simulink model "ClimbSim"  (R2022a)
settings: Solver=VariableStepAuto  StartTime=0.0  StopTime=inf  RelTol=1e-3
values from neighbouring files (symbols this model uses):
  EMFCoefCim = 18.803/1000    (= 0.018803)    [Climbing.m]    (also in Launch.m; Launching.m)
  InputClimbing = 1    [Climbing.m]    (also in Launching.m)
  loadInertiaClimbing = 6.12 / (2*12.75) + (1.27*0.6*(0.0254^2))/2    (= 0.24024580596)    [Climbing.m]    (also in Launching.m)
  LVDTGain = 0.0084*1000    (= 8.4)    [Climbing.m]
  LVDTOffset = 0.0105    [Climbing.m]
  mechDampingConstantClimbing = (TorqueCoefCim * EMFCoefCim) / TerminalResistanceCim    (= 0.000117850936333)    [Climbing.m]    (also in Launching.m)
  TerminalInductanceCim = 122/1000000    (= 0.000122)    [Climbing.m]    (also in Launch.m; Launching.m)
  TerminalResistanceCim = 3    [Climbing.m]    (also in Launch.m; Launching.m)
  TorqueCoefCim = 18.803/1000    (= 0.018803)    [Climbing.m]    (also in Launch.m; Launching.m)
  TorqueDisturbanceClimb = 0    [Climbing.m]
libraries: slpidlib x1
settings Model: PacingRate=1.100000  Creator=JD Herlehy  LastModifiedBy=JD Herlehy

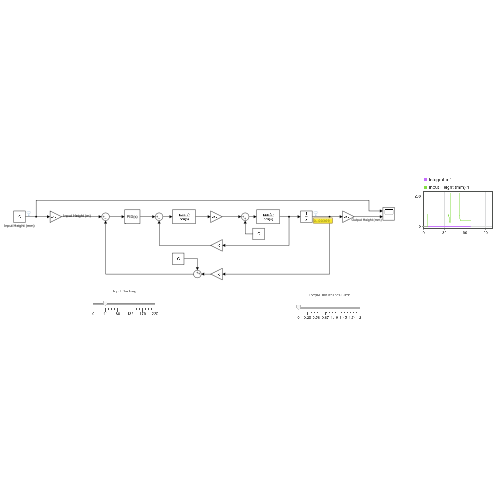
[thumbnail: Simulink's stored preview of the top-level diagram]
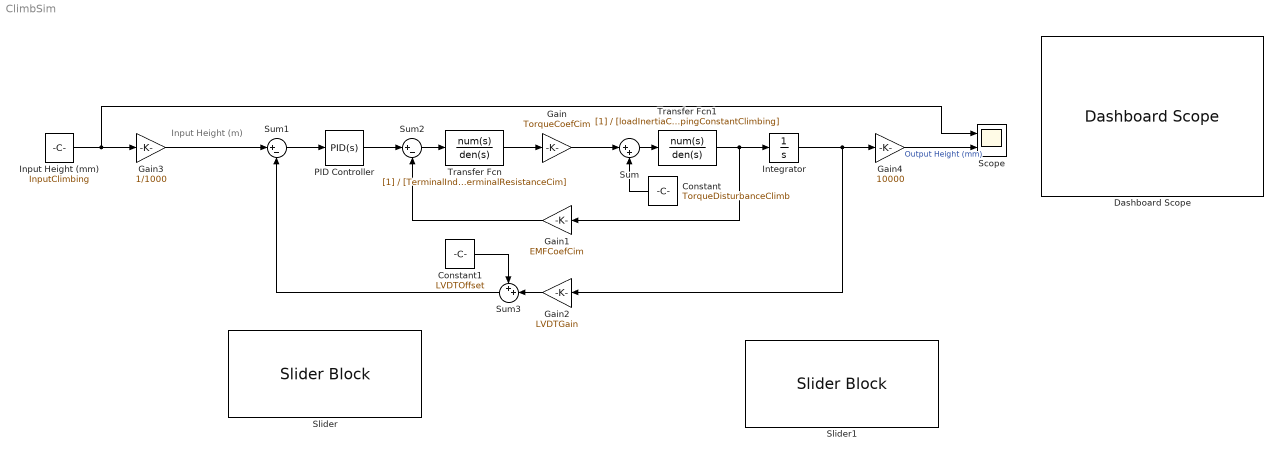
== system ClimbSim ==
  note: Input Height (m)
  Constant : Constant  Value=TorqueDisturbanceClimb
  Constant1 : Constant  Value=LVDTOffset
  Dashboard Scope : DashboardScope  Ymin=-5  Ymax=420
  Gain : Gain  Gain=TorqueCoefCim
  Gain1 : Gain  Gain=EMFCoefCim
  Gain2 : Gain  Gain=LVDTGain
  Gain3 : Gain  Gain=1/1000
  Gain4 : Gain  Gain=10000
  Input Height (mm) : Constant  Value=InputClimbing
  Integrator : Integrator
  PID Controller : slpidlib/PID Controller  Controller=PID  Form=Parallel  TimeDomain=Continuous-time  UseExternalTs=off  SampleTime=-1  IntegratorMethod=Forward Euler  FilterMethod=Forward Euler  ControllerParametersSource=internal  P=0.119769025482239  I=0.000698723978175495  UseKiTs=off  D=4.56146509375894  N=114.28279760416  UseFilter=on  TunerSelectOption=Transfer Function Based (PID Tuner App)  InitialConditionSource=internal  InitialConditionForIntegrator=0  InitialConditionForFilter=0  DifferentiatorICPrevScaledInput=0  ExternalReset=none  TrackingMode=off  Kt=1  LimitOutput=off  SatLimitsSource=internal  UpperSaturationLimit=inf  LowerSaturationLimit=-inf  LinearizeAsGain=on  AntiWindupMode=none  Kb=1  POutMin=[]  POutMax=[]  IOutMin=[]  IOutMax=[]  DOutMin=[]  DOutMax=[]  NOutMin=[]  NOutMax=[]  SumOutMin=[]  SumOutMax=[]  SaturationOutMin=[]  SaturationOutMax=[]  PParamMin=[]  PParamMax=[]  IParamMin=[]  IParamMax=[]  DParamMin=[]  DParamMax=[]  NParamMin=[]  NParamMax=[]  KbParamMin=[]  KbParamMax=[]  KtParamMin=[]  KtParamMax=[]  KbOutMin=[]  KbOutMax=[]  KtOutMin=[]  KtOutMax=[]  IntegratorOutMin=[]  IntegratorOutMax=[]  FilterOutMin=[]  FilterOutMax=[]  SumI1OutMin=[]  SumI1OutMax=[]  SumI2OutMin=[]  SumI2OutMax=[]  SumI3OutMin=[]  SumI3OutMax=[]  SumI4OutMin=[]  SumI4OutMax=[]  SumDOutMin=[]  SumDOutMax=[]  DifferentiatorOutMin=[]  DifferentiatorOutMax=[]  FilterDiffOutCoefMin=[]  FilterDiffOutCoefMax=[]  ReciprocalOutMin=[]  ReciprocalOutMax=[]  SumDenOutMin=[]  SumDenOutMax=[]  SumNumOutMin=[]  SumNumOutMax=[]  DivideOutMin=[]  DivideOutMax=[]  UdiffTsProdOutMin=[]  UdiffTsProdOutMax=[]  NTsProdOutMin=[]  NTsProdOutMax=[]  UintegralTsProdOutMin=[]  UintegralTsProdOutMax=[]  UngainTsProdOutMin=[]  UngainTsProdOutMax=[]  IntegratorContinuousStateAttributes=''  IntegratorStateMustResolveToSignalObject=off  IntegratorRTWStateStorageClass=Auto  FilterContinuousStateAttributes=''  FilterStateMustResolveToSignalObject=off  FilterRTWStateStorageClass=Auto  ParallelPVariant=InternalParameters  IdealPVariant=Disabled  IVariant=InternalParameters  DVariant=InternalParameters  IntegratorVariant=Continuous  SatVariant=Disabled  AWVariant=Passthrough  PCopyVariant=Disabled  TRVariant=Disabled  FdbkBlocksVariant=Forward  IdealPFdbkVariant=Disabled  SatFdbkVariant=Disabled  DerivativeFilterVariant=ContFilter  NVariant=InternalParameters  NCopyVariant=Disabled  FilterICVariant=InternalICsFilter  IntegratorICVariant=InternalICs  ExternalResetVariant=Disabled  TRSumVariant=Passthrough  SumFdbkVariant=Disabled  SumVariant=Sum_PID  TsampFilterVariant=InternalTs  TsampNgainVariant=Passthrough  TsampIntegralVariant=Passthrough  ExternalSaturationOutDataTypeStr=Inherit: Same as second input  aMode=0
  Scope : Scope  NumInputPorts=2
  Slider : SliderBlock  ScaleMax=220
  Slider1 : SliderBlock  ScaleMax=2
  Sum : Sum  Inputs=|++
  Sum1 : Sum  Inputs=|+-
  Sum2 : Sum  Inputs=|+-
  Sum3 : Sum  Inputs=++|
  Transfer Fcn : TransferFcn  Denominator=[TerminalInductanceCim TerminalResistanceCim]
  Transfer Fcn1 : TransferFcn  Denominator=[loadInertiaClimbing mechDampingConstantClimbing]
  wires:
  Transfer Fcn1/1 -> Gain1/1, Integrator/1
  Integrator/1 -> Gain2/1, Gain4/1
  Gain1/1 -> Sum2/2
  Transfer Fcn/1 -> Gain/1
  Sum/1 -> Transfer Fcn1/1
  Constant/1 -> Sum/2
  Sum2/1 -> Transfer Fcn/1
  Gain/1 -> Sum/1
  Gain2/1 -> Sum3/2
  Constant1/1 -> Sum3/1
  Sum3/1 -> Sum1/2
  Input Height (mm)/1 -> Scope/1, Gain3/1
  Gain4/1 -> Scope/2  "Output Height (mm)"
  Sum1/1 -> PID Controller/1
  Gain3/1 -> Sum1/1
  PID Controller/1 -> Sum2/1
